simulink model "Ejemplo03"  (R2021b)
settings: Solver=VariableStepAuto  StartTime=0.0  StopTime=200  MaxStep=0.001  RelTol=1e-3
settings Model: Creator=juandiegocastropadilla  LastModifiedBy=juandiegocastropadilla

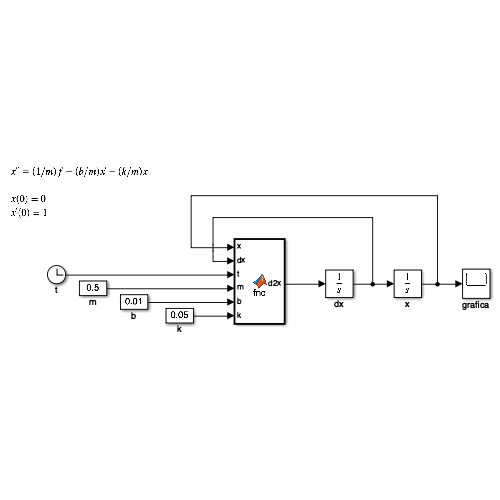
[thumbnail: Simulink's stored preview of the top-level diagram]
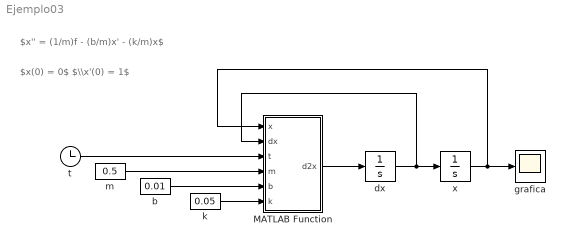
== system Ejemplo03 ==
  note: $x'' = (1/m)f - (b/m)x' - (k/m)x$
  note: $x(0) = 0$ $\\x'(0) = 1$
  MATLAB Function : MATLAB Function  TreatAsAtomicUnit=on
  b : Constant  Value=0.01
  dx : Integrator  InitialCondition=1
  grafica : Scope
  k : Constant  Value=0.05
  m : Constant  Value=0.5
  t : Clock
  x : Integrator
  wires:
  MATLAB Function/1(d2x) -> dx/1
  dx/1 -> x/1, MATLAB Function/2(dx)
  x/1 -> grafica/1, MATLAB Function/1(x)
  t/1 -> MATLAB Function/3(t)
  m/1 -> MATLAB Function/4(m)
  b/1 -> MATLAB Function/5(b)
  k/1 -> MATLAB Function/6(k)

== matlab function Ejemplo03/MATLAB Function ==
  data: x input; d2x output; dx input; t input; m input; b input; k input
function d2x = fnc(x, dx, t, m, b, k)

f = t;

d2x = ((1/m)*f - (b/m)*dx - (k/m)*x);
